simulink model "state_space_model"  (R2022b)
settings: Solver=VariableStepAuto  StartTime=0.0  StopTime=10.0  RelTol=1e-3
undefined symbols (not defined in the file or in its folder): A6, B6, C6, D6, E5, F5
settings Model: Creator=ramuj  LastModifiedBy=USUARIO

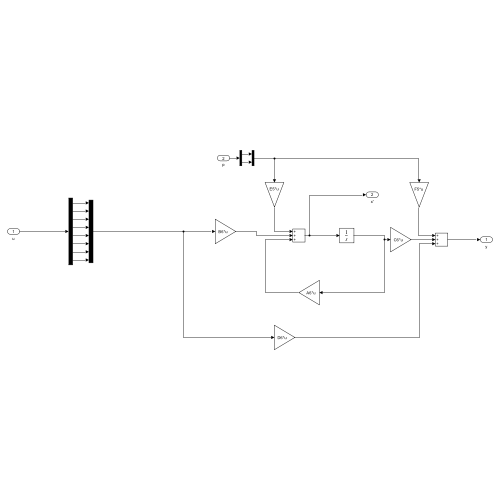
[thumbnail: Simulink's stored preview of the top-level diagram]
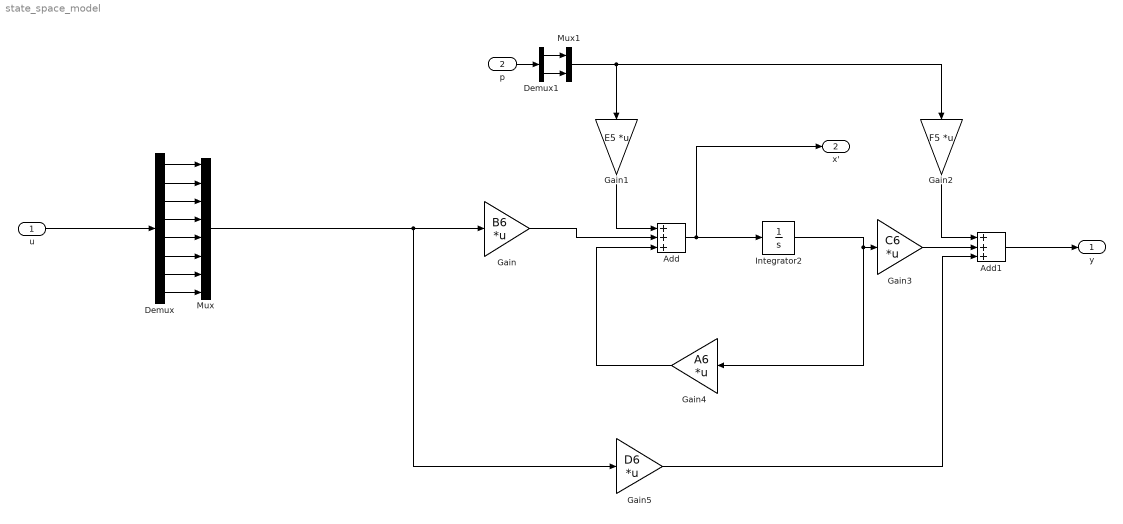
== system state_space_model ==
  u : Inport
  p : Inport  Port=2
  Add : Sum  Inputs=+++
  Add1 : Sum  Inputs=+++
  Demux : Demux  Outputs=8
  Demux1 : Demux  Outputs=2
  Gain : Gain  Gain=B6  Multiplication=Matrix(K*u)
  Gain1 : Gain  Gain=E5  Multiplication=Matrix(K*u)
  Gain2 : Gain  Gain=F5  Multiplication=Matrix(K*u)
  Gain3 : Gain  Gain=C6  Multiplication=Matrix(K*u)
  Gain4 : Gain  Gain=A6  Multiplication=Matrix(K*u)
  Gain5 : Gain  Gain=D6  Multiplication=Matrix(K*u)
  Integrator2 : Integrator
  Mux : Mux  Inputs=8
  Mux1 : Mux  Inputs=2
  y : Outport
  x' : Outport  Port=2
  wires:
  Mux1/1 -> Gain2/1, Gain1/1
  Gain1/1 -> Add/1
  Gain/1 -> Add/2
  Add/1 -> Integrator2/1, x'/1
  Integrator2/1 -> Gain4/1, Gain3/1
  Gain3/1 -> Add1/2
  Gain2/1 -> Add1/1
  Add1/1 -> y/1
  Gain4/1 -> Add/3
  Gain5/1 -> Add1/3
  Mux/1 -> Gain5/1, Gain/1
  u/1 -> Demux/1
  Demux/1 -> Mux/1
  Demux/2 -> Mux/2
  Demux/3 -> Mux/3
  Demux/4 -> Mux/4
  Demux/5 -> Mux/5
  Demux/6 -> Mux/6
  Demux/7 -> Mux/7
  Demux/8 -> Mux/8
  Demux1/1 -> Mux1/1
  Demux1/2 -> Mux1/2
  p/1 -> Demux1/1
